simulink model "fixed_speed_turbine_simulation"  (R2023a)
settings: Solver=ode45  StartTime=0.0  StopTime=simtime  MaxStep=0.1e-3  RelTol=1e-3
values from neighbouring files (symbols this model uses):
  angle_pitch = angle_pitch+0.1    (= 0.1)    [fix_speed_ss_model_Tasos_WITHOUT_CP_LIMITING.m]    (also in fixed_speed_turbine_script.m = 0; steady_state_squirrel_cage_im_operation_points.m = 0)
  Area_swept_by_the_blades = pi*rotor_radius^2    (= 4536.45979178)    [fix_speed_ss_model_Tasos_WITHOUT_CP_LIMITING.m]    (also in fixed_speed_turbine_script.m)
  grid_freq = 50    [fix_speed_ss_model_Tasos_WITHOUT_CP_LIMITING.m]    (also in fixed_speed_turbine_script.m)
  moment_of_inertia = 90    [fix_speed_ss_model_Tasos_WITHOUT_CP_LIMITING.m]    (also in fixed_speed_turbine_script.m)
  nominal_voltage = 960    [fix_speed_ss_model_Tasos_WITHOUT_CP_LIMITING.m]    (also in fixed_speed_turbine_script.m)
  pole_pairs = 2    [fix_speed_ss_model_Tasos_WITHOUT_CP_LIMITING.m]    (also in fixed_speed_turbine_script.m)
  rho = 1.225    [anthony_ode_FINALCODESteady.m]    (also in fix_speed_ss_model_Tasos_WITHOUT_CP_LIMITING.m; fixed_speed_turbine_script.m; steady_state.m; steady_state_squirrel_cage_im_operation_points.m)
  rotor_leakage_inductance = 3e-4    (= 0.0003)    [fix_speed_ss_model_Tasos_WITHOUT_CP_LIMITING.m]    (also in fixed_speed_turbine_script.m)
  rotor_radius = rotor_diameter/2    (= 38)    [fix_speed_ss_model_Tasos_WITHOUT_CP_LIMITING.m]    (also in fixed_speed_turbine_script.m)
  rotor_resistance = 0.009    [fix_speed_ss_model_Tasos_WITHOUT_CP_LIMITING.m]    (also in fixed_speed_turbine_script.m)
  simtime = 10    [fixed_speed_turbine_script.m]
  stator_leakage_inductance = 4e-4    (= 0.0004)    [fix_speed_ss_model_Tasos_WITHOUT_CP_LIMITING.m]    (also in fixed_speed_turbine_script.m)
  stator_resistance = 0.005    [fix_speed_ss_model_Tasos_WITHOUT_CP_LIMITING.m]    (also in fixed_speed_turbine_script.m)
  transmission_ratio = 80    [fix_speed_ss_model_Tasos_WITHOUT_CP_LIMITING.m]    (also in fixed_speed_turbine_script.m)
  tsr = 0:.1:20    [fix_speed_ss_model_Tasos_WITHOUT_CP_LIMITING.m]    (also in fixed_speed_turbine_script.m = 0:.1:17; steady_state_squirrel_cage_im_operation_points.m = w2*R_turbina/(n_multiplicador*vw))
  w_ini = 2*pi*grid_freq/(pole_pairs* transmission_ratio)    (= 1.96349540849)    [fix_speed_ss_model_Tasos_WITHOUT_CP_LIMITING.m]    (also in fixed_speed_turbine_script.m)
undefined symbols (not defined in the file or in its folder): ArrayofCp
libraries: simulink x3, spsAsynchronousMachineSIUnitsLib x1, spsGroundLib x1, spsPower3phInstantaneousLib x1, spsRMSLib x1, eeStairGenerator x1, spsThreePhaseProgrammableVoltageSourceLib x1, spsThreePhaseVIMeasurementLib x1, spspowerguiLib x1
settings Model: Creator=citcea  LastModifiedBy=citcea

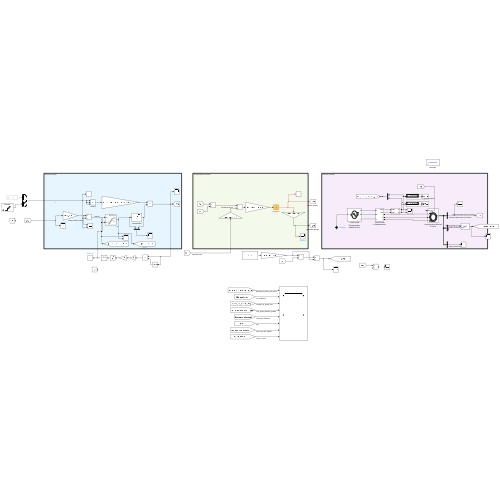
[thumbnail: Simulink's stored preview of the top-level diagram]
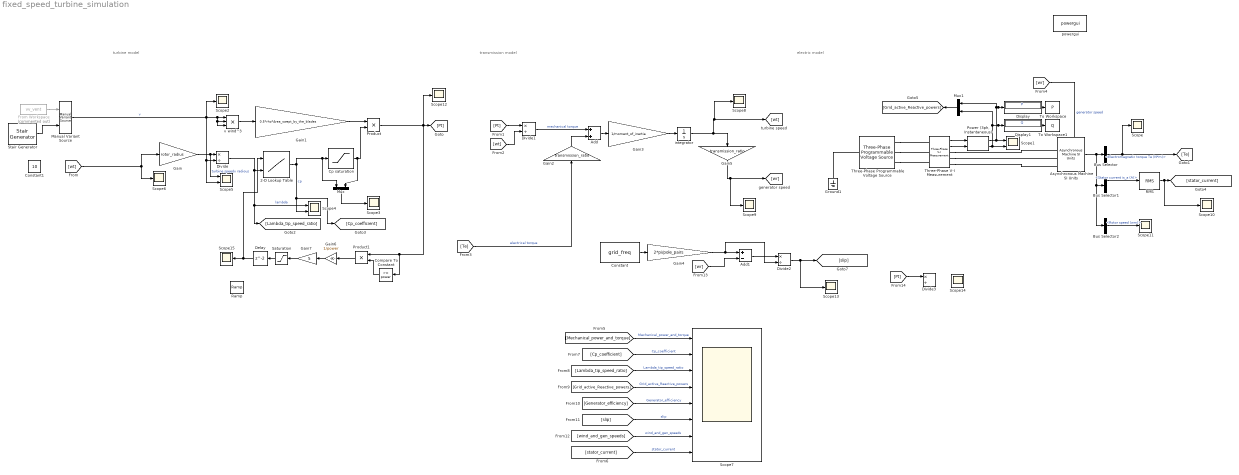
== system fixed_speed_turbine_simulation ==
  note: turbine model
  note: transmission model
  note: electric model
  2-D Lookup Table : Lookup_n-D  BreakpointsForDimension1=angle_pitch  BreakpointsForDimension2=tsr  Table=ArrayofCp  InternalRulePriority=Speed  RndMeth=Simplest
      settings: InputPortMap=u0,u1
  Add : Sum
  Add1 : Sum  Inputs=+-
  "Asynchronous Machine SI Units " : spsAsynchronousMachineSIUnitsLib/Asynchronous Machine SI Units  RotorType=Squirrel-cage  PresetModel=No  MechanicalLoad=Speed w  ShowDetailedParameters=on  ReferenceFrame=Rotor  Units=SI  MeasurementBus=off  NominalParameters=[power nominal_voltage grid_freq]  VoltageRatio=1  Stator=[stator_resistance stator_leakage_inductance]  Rotor=[rotor_resistance rotor_leakage_inductance]  Cage1=[0.4155 0.002066]  Cage2=[0.4168 0.0003495]  Lm=magnetizing_inductance  Mechanical=[0.05 0.005879 pole_pairs]  PolePairs=pole_pairs  InitialConditions=[0.01 0 0 0 0 0 0 0]  SimulateSaturation=off  Saturation=[14.03593122, 27.81365428, 53.79336849, 72.68890987, 97.98006896, 148.6815601, 215.7428561, 302.9841135, 428.7778367 ; 230, 322, 414, 460, 506, 552, 598, 644, 690]  LoadFlowParameters=1492000  TsPowergui=0  TsBlock=-1  IterativeModel=Trapezoidal non iterative  IterativeDiscreteModel=Trapezoidal non iterative  Pmec=1.492e+006
  Bus Selector : BusSelector  OutputSignals=Mechanical.Electromagnetic torque Te (N*m)
  Bus Selector1 : BusSelector  OutputSignals=Stator measurements.Stator current is_a (A),Stator measurements.Stator current is_b (A),Stator measurements.Stator current is_c (A)
  Bus Selector2 : BusSelector  OutputSignals=Mechanical.Rotor speed (wm)
  Compare To Constant : simulink/Logic and Bit Operations/Compare To Constant  relop=>=  const=power  OutDataTypeStr=boolean
  Constant : Constant  Value=grid_freq
  Constant1 : Constant  Value=10
  Cp saturation : Saturate
  Delay : Delay
  Display : Display
  Display1 : Display
  Divide{,1..3} (4 alike) : Product  Inputs=*/
  From Workspace : FromWorkspace  Commented=on  VariableName=vv_vent
  Gain : Gain  Gain=rotor_radius
  Gain1 : Gain  Gain=0.5*rho*Area_swept_by_the_blades
  Gain2 : Gain  Gain=transmission_ratio
  Gain3 : Gain  Gain=1/moment_of_inertia
  Gain4 : Gain  Gain=2*pi/pole_pairs
  Gain5 : Gain  Gain=transmission_ratio
  Gain6 : Gain  Gain=1/power
  Gain7 : Gain  Gain=5
  Ground1 : spsGroundLib/Ground  LConnTagsString=a
  Manual Variant Source : simulink/Signal Routing/Manual Variant Source  NumChoices=2  LabelModeActiveChoice=V_2
  Mux : Mux  Inputs=2
  Mux1 : Mux  Inputs=2
  "Power (3ph, Instantaneous)" : spsPower3phInstantaneousLib/Power (3ph, Instantaneous)
  Product : Product
  Product1 : Product
  RMS : spsRMSLib/RMS  TrueRMS=on  Freq=grid_freq  RMSInit=0  Ts=0
  Ramp : simulink/Sources/Ramp  slope=1  start=0  InitialOutput=0
  Saturation : Saturate  UpperLimit=2*17  LowerLimit=0
  Scope{,2..3,6,8..15} (12 alike) : Scope
  Scope1 : Scope  NumInputPorts=2
  Scope4 : Scope  NumInputPorts=2
  Scope5 : Scope  NumInputPorts=2
  Scope7 : Scope  NumInputPorts=8
  Stair Generator : eeStairGenerator/Stair Generator  LabelModeActiveChoice=Discrete  TimeInput=[0 simtime/4 2*(simtime/4) 3*(simtime/4) simtime]  AmplitudeInput=[ 7 7 11 14 14]  SampleTime=simtime/100  RepeatPattern=off  OutDataTypeStr=double
      settings: LibrarySourceBlock=ee_sl_lib/General Control/Stair Generator
  "Three-Phase Programmable Voltage Source " : spsThreePhaseProgrammableVoltageSourceLib/Three-Phase Programmable Voltage Source  PositiveSequence="[nominal_voltage  0 grid_freq]"  VariationEntity=None  VariationType=Table of time-amplitude pairs  VariationTypeAlt=Step  VariationStep=0.5  VariationRate=10  VariationMagnitude=0.3  VariationFrequency=2  VariationTiming=[1 2]  VariationPhaseA=off  Amplitudes=[1 0.8 1.2 1.0]  TimeValues=[0 0.1 0.15 0.2]  HarmonicGeneration=off  HarmonicA=[3 0.2 -25 0]  HarmonicB=[2 0.15 35 2]  Timing="[0.05  3]"  BusType=swing  Pref=0  Qref=0  Qmin=-inf  Qmax=inf
  "Three-Phase V-I Measurement " : spsThreePhaseVIMeasurementLib/Three-Phase V-I Measurement  VoltageMeasurement=phase-to-ground  SetLabelV=off  LabelV=Vabc  Vpu=off  VpuLL=off  CurrentMeasurement=yes  SetLabelI=off  LabelI=Iabc  Ipu=off  Pbase=100e6  Vbase=500e3  OutputType=Complex  PhasorSimulation=off  PSBequivalent=0
  To Workspace : ToWorkspace  VariableName=P  SaveFormat=Timeseries  SampleTime=-1
  To Workspace1 : ToWorkspace  VariableName=Q  SaveFormat=Timeseries  SampleTime=-1
  integrator : Integrator  InitialCondition=w_ini  UpperSaturationLimit=w_ini*100  LowerSaturationLimit=-w_ini*100
  powergui : spspowerguiLib/powergui  Priority=1  SimulationMode=Continuous  SampleTime=50e-6  frequency=60  Iterations=50  frequencyindice=50  Pbase=100e6  ErrMax=1e-4  UnitsV=kV  UnitsW=MW  buscounter=0  FunctionMessages=off  echomessages=off  EnableUseOfTLC=off  CurrentSourceSwitches=off  DisableSnubberDevices=off  DisableRonSwitches=off  DisableVfSwitches=off  DisplayEquations=off  AutomaticDiscreteSolvers=off  SolverType=Tustin/Backward Euler (TBE)  Interpol=off  ExternalGateDelay=off  methode=off  Ts=100  x0status=blocks  SPID=on  SwTol=0  HookPort=off  NonlinearTolerance=1e-4  nMaxIteration=100  ContinueOnMaxIteration=off  RestoreLinks=warning  ResistiveCurrentMeasurement=off  Frange=[0:2:500]  Ylog=off  Xlog=on  ShowGrid=off  save=off  variable=ZData  structure=0  ZoomFFT=off  StartTime=0.0  cycles=1  DisplayStyle=1  fundamental=60  FreqAxis=off  MaxFrequency=1000  frequencyindicesteady=1  RmsSteady=1  display=off
  v wind^3 : Product  Inputs=3
  wires:
  Gain/1 -> Scope5/1, Divide/1  "turbine speedx radious"
  Manual Variant Source/1 -> Scope2/1, v wind^3/3, v wind^3/2, v wind^3/1, Scope5/2, Divide/2  "v"
  v wind^3/1 -> Gain1/1
  Gain1/1 -> Product/1
  Cp saturation/1 -> Mux/2, Product/2
  2-D Lookup Table/1 -> Mux/1, Cp saturation/1, [Cp_coefficient], Scope4/2  "cp"
  [Pt] -> Divide1/1
  [wt] -> Divide1/2
  Divide1/1 -> Add/1  "mechanical torque"
  Gain2/1 -> Add/2
  [Te] -> Gain2/1  "electrical torque"
  Add/1 -> Gain3/1
  Gain3/1 -> integrator/1
  integrator/1 -> Gain5/1, Scope8/1, [wt]
  Gain5/1 -> Scope9/1, [wr]
  "Three-Phase V-I Measurement "/1 -> "Power (3ph, Instantaneous)"/1
  "Three-Phase V-I Measurement "/2 -> "Power (3ph, Instantaneous)"/2
  [wr] -> "Asynchronous Machine SI Units "/1  "generator speed"
  "Asynchronous Machine SI Units "/1 -> Bus Selector2/1, Bus Selector1/1, Bus Selector/1
  Bus Selector/1 -> Scope/1, [Te]  "<Electromagnetic torque Te (N*m)>"
  From Workspace/1 -> Manual Variant Source/1
  Stair Generator/1 -> Manual Variant Source/2
  "Power (3ph, Instantaneous)"/2 -> Mux1/2, To Workspace1/1, Display1/1, Scope1/2  "Q"
  "Power (3ph, Instantaneous)"/1 -> Mux1/1, Display/1, To Workspace/1, Scope1/1  "P"
  Mux/1 -> Scope3/1
  Divide/1 -> 2-D Lookup Table/2, [Lambda_tip_speed_ratio], Scope4/1  "lambda"
  [Mechanical_power_and_torque] -> Scope7/1  "Mechanical_power_and_torque"
  [Cp_coefficient] -> Scope7/2  "Cp_coefficient"
  [Lambda_tip_speed_ratio] -> Scope7/3  "Lambda_tip_speed_ratio"
  [Grid_active_Reactive_powers] -> Scope7/4  "Grid_active_Reactive_powers"
  [Generator_efficiency] -> Scope7/5  "Generator_efficiency"
  [slip] -> Scope7/6  "slip"
  [wind_and_gen_speeds] -> Scope7/7  "wind_and_gen_speeds"
  [stator_current] -> Scope7/8  "stator_current"
  Bus Selector1/1 -> RMS/1  "<Stator current is_a (A)>"
  Mux1/1 -> [Grid_active_Reactive_powers]
  Divide2/1 -> Scope13/1, [slip]
  [wr] -> Add1/2
  Constant/1 -> Gain4/1
  Gain4/1 -> Divide2/2, Add1/1
  Add1/1 -> Divide2/1
  RMS/1 -> Scope10/1, [stator_current]
  Bus Selector2/1 -> Scope11/1  "<Rotor speed (wm)>"
  [Pt] -> Divide3/1
  [wt] -> Gain/1, Scope6/1
  Delay/1 -> 2-D Lookup Table/1, Scope15/1
  Gain6/1 -> Gain7/1
  Gain7/1 -> Saturation/1
  Saturation/1 -> Delay/1
  Product/1 -> Compare To Constant/1, Product1/1, Scope12/1, [Pt]
  Compare To Constant/1 -> Product1/2
  Product1/1 -> Gain6/1
  connections:
  "Three-Phase Programmable Voltage Source "/RConn1 -- "Three-Phase V-I Measurement "/LConn1
  "Three-Phase Programmable Voltage Source "/RConn2 -- "Three-Phase V-I Measurement "/LConn2
  "Three-Phase Programmable Voltage Source "/RConn3 -- "Three-Phase V-I Measurement "/LConn3
  "Three-Phase V-I Measurement "/RConn3 -- "Asynchronous Machine SI Units "/LConn3
  "Three-Phase V-I Measurement "/RConn2 -- "Asynchronous Machine SI Units "/LConn2
  "Three-Phase V-I Measurement "/RConn1 -- "Asynchronous Machine SI Units "/LConn1
  Ground1/LConn1 -- "Three-Phase Programmable Voltage Source "/LConn1
